simulink model "Gois09"  (R2023b)
settings: Solver=VariableStepAuto  StartTime=t(1)  StopTime=t(end)  FixedStep=dt  RelTol=1e-3
values from neighbouring files (symbols this model uses):
  params = [ ... (first row only)    [gois09_simulink.m]    (also in ryzhii14_simulink.m; sinoatrial_simulink.m; vdp_simulink.m)
  xInitial = [initial_conditions ... (first row only)    [gois09_simulink.m]    (also in hilaire07martinez_simulink.m = initial_conditions(1:2); jewett99_simulink.m = initial_conditions(1:2); ryzhii14_simulink.m; sinoatrial_simulink.m = initial_conditions)
settings Model: Creator=chukw  LastModifiedBy=chukw

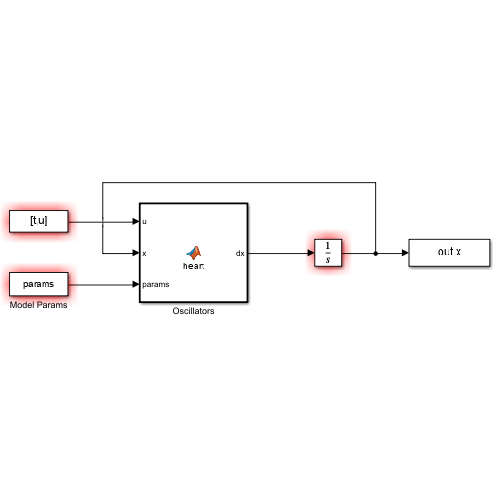
[thumbnail: Simulink's stored preview of the top-level diagram]
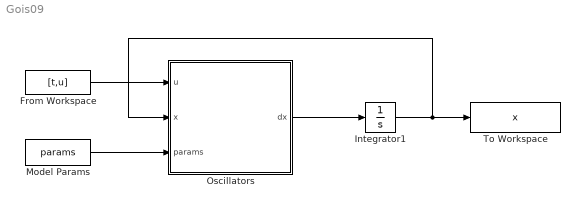
== system Gois09 ==
  From Workspace : FromWorkspace  VariableName=[t,u]
  Integrator1 : Integrator  InitialCondition=xInitial
  Model Params : Constant  Value=params
  Oscillators : MATLAB Function  TreatAsAtomicUnit=on
  To Workspace : ToWorkspace  VariableName=x  SampleTime=-1
  wires:
  Integrator1/1 -> Oscillators/2(x), To Workspace/1
  Oscillators/1(dx) -> Integrator1/1
  Model Params/1 -> Oscillators/3(params)
  From Workspace/1 -> Oscillators/1(u)

== matlab function Gois09/Oscillators ==
  data: u input; dx output; x input; params input
function dx = heart(u, x, params)
    % Sino-Atrial parameters.
    a_sa = params(1);
    w_sa1 = params(2);
    w_sa2 = params(3);
    d_sa = params(4);
    e_sa = params(5);

    % Atrio-Ventricular parameters.
    a_av = params(6);
    w_av1 = params(7);
    w_av2 = params(8);
    d_av = params(9);
    e_av = params(10);

    % His-Purkinje complex parameters.
    a_hp = params(11);
    w_hp1 = params(12);
    w_hp2 = params(13);
    d_hp = params(14);
    e_hp = params(15);

    % ECG parameters.
    alf_0 = params(16);
    alf_1 = params(17);
    alf_3 = params(18);
    alf_5 = params(19);

    % Coupling parameters.
    k_sa_av = params(20);
    k_sa_hp = params(21);
    k_av_sa = params(22);
    k_av_hp = params(23);
    k_hp_sa = params(24);
    k_hp_av = params(25);

    % Differential equations.
    dx = zeros(7, 1);

    % SA Node.
    dx(1) = x(2);
    dx(2) = (-a_sa*x(2)*(x(1) - w_sa1)*(x(1) - w_sa2)) -...
        (x(1)*(x(1) + d_sa)*(x(1) + e_sa)) + (k_sa_av*(x(1) - x(3))) +...
        (k_sa_hp*(x(1) - x(5)));

    % AV Node.
    dx(3) = x(4);
    dx(4) = (-a_av*x(4)*(x(3) - w_av1)*(x(3) - w_av2)) -...
        (x(3)*(x(3) + d_av)*(x(3) + e_av)) + (k_av_sa*(x(3) - x(1))) +...
        (k_av_hp*(x(3) - x(5)));

    % HP Complex.
    dx(5) = x(6);
    dx(6) = (-a_hp*x(6)*(x(5) - w_hp1)*(x(5) - w_hp2)) -...
        (x(5)*(x(5) + d_hp)*(x(5) + e_hp)) + (k_hp_sa*(x(5) - x(1))) +...
        (k_hp_av*(x(5) - x(3)));

    % ECG.
    dx(7) = (alf_1*x(2)) + (alf_3*x(4)) + (alf_5*x(6));
end
